simulink model "untitled"  (Simulink 4.00)
settings: Solver=ode45  StartTime=0.0  StopTime=10.0  RelTol=1e-3
settings Model: LastModifiedBy=aluno

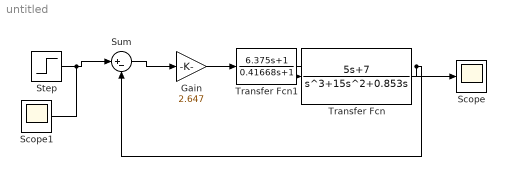
== system untitled ==
  Gain : Gain  Gain=2.647  Multiplication=Element-wise(K.*u)  SaturateOnIntegerOverflow=on
  Scope : Scope
      settings: TimeRange=auto  YMin=-5  YMax=5  SaveToWorkspace=off  SaveName=ScopeData  LimitDataPoints=on  MaxDataPoints=5000
  Scope1 : Scope
      settings: TimeRange=auto  YMin=-5  YMax=5  SaveToWorkspace=off  LimitDataPoints=on  MaxDataPoints=5000
  Step : Step  Time=0  Before=0  After=1  SampleTime=0
  Sum : Sum  Inputs=|+-  SaturateOnIntegerOverflow=on
  Transfer Fcn : TransferFcn  Numerator=[5 7]  Denominator=[1 15 0.853 0]  AbsoluteTolerance=auto  Realization=auto
  Transfer Fcn1 : TransferFcn  Numerator=[6.375 1]  Denominator=[0.41668 1]  AbsoluteTolerance=auto  Realization=auto
  wires:
  Transfer Fcn/1 -> Scope/1, Sum/2
  Transfer Fcn1/1 -> Transfer Fcn/1
  Gain/1 -> Transfer Fcn1/1
  Sum/1 -> Gain/1
  Step/1 -> Sum/1, Scope1/1
